simulink model "rfdc"  (R2019a)
settings: Solver=VariableStepAuto  StartTime=0.0  StopTime=10.0  RelTol=1e-3
libraries: xbsIndex_r4 x4
settings Model: Creator=mcb  LastModifiedBy=mcb

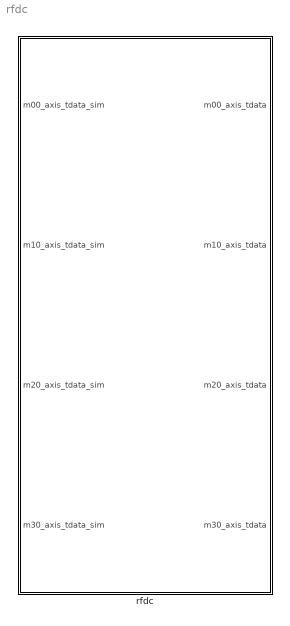
== system rfdc ==
  rfdc : Subsystem  Tag=xps:rfdc  mask(Xilinx RF Data Converter){Tile224_enable=on, Tile225_enable=on, Tile226_enable=on, Tile227_enable=on, enable_mts=off, sample_rate=2000, clk_out=250, enable_pll=on, ref_clk=250, axi_stream_clk=[], QT_adc0_enable=on, QT_adc0_digital_output=Real, QT_adc0_dec_mode=8x, QT_adc0_sample_per_cycle=1, QT_adc0_req_axis_clk=250, QT_adc0_mixer_type=Bypassed, QT_adc0_mixer_mode=Real -> Real, QT_adc0_nco_freq=0, QT_adc0_nco_phase=0, QT_adc0_coarse_freq=0, QT_adc0_nyquist_zone=Zone 1, QT_adc0_cal_mode=Mode 2, QT_adc1_enable=off, QT_adc1_digital_output=Real, QT_adc1_dec_mode=1x, QT_adc1_sample_per_cycle=4, QT_adc1_req_axis_clk=500, QT_adc1_mixer_type=Bypassed, QT_adc1_mixer_mode=Real -> Real, QT_adc1_nco_freq=0, QT_adc1_nco_phase=0, QT_adc1_coarse_freq=0, QT_adc1_nyquist_zone=Zone 2, QT_adc1_cal_mode=Mode 2, QT_adc2_enable=off, QT_adc2_digital_output=Real, QT_adc2_dec_mode=8x, QT_adc2_sample_per_cycle=1, QT_adc2_req_axis_clk=250, QT_adc2_mixer_type=Bypassed, QT_adc2_mixer_mode=Real -> Real, QT_adc2_nco_freq=0, QT_adc2_nco_phase=0, QT_adc2_coarse_freq=0, QT_adc2_nyquist_zone=Zone 1, QT_adc2_cal_mode=Mode 2, QT_adc3_enable=off, QT_adc3_digital_output=Real, QT_adc3_dec_mode=8x, QT_adc3_sample_per_cycle=1, QT_adc3_req_axis_clk=250, QT_adc3_mixer_type=Bypassed, QT_adc3_mixer_mode=Real -> Real, QT_adc3_nco_freq=0, QT_adc3_nco_phase=0, QT_adc3_coarse_freq=0, QT_adc3_nyquist_zone=Zone 1, QT_adc3_cal_mode=Mode 2, DT_adc0_enable=on, DT_adc0_digital_output=Real, DT_adc0_dec_mode=2x, DT_adc0_sample_per_cycle=8, DT_adc0_req_axis_clk=0, DT_adc0_mixer_type=Bypassed, DT_adc0_mixer_mode=Real -> Real, DT_adc0_nco_freq=0, DT_adc0_nco_phase=0, DT_adc0_coarse_freq=Fs/2, DT_adc0_nyquist_zone=Zone 1, DT_adc0_cal_mode=Mode 2, DT_adc1_enable=on, DT_adc1_digital_output=Real, DT_adc1_dec_mode=2x, DT_adc1_sample_per_cycle=8, DT_adc1_req_axis_clk=0, DT_adc1_mixer_type=Bypassed, DT_adc1_mixer_mode=Real -> Real, DT_adc1_nco_freq=0, DT_adc1_nco_phase=0, DT_adc1_coarse_freq=Fs/2, DT_adc1_nyquist_zone=Zone 1, DT_adc1_cal_mode=Mode 2}
      mask prompts: Tile224_enable "Tile 224"; Tile225_enable "Tile 225"; Tile226_enable "Tile 226"; Tile227_enable "Tile 227"; enable_mts "Enable Multi-Tile Sync"; sample_rate "Sampling Rate (Msps)"; clk_out "Clock Out (MHz)"; enable_pll "Enable Tile PLLs"; ref_clk "Reference Clock (MHz)"; axi_stream_clk "Required AXI4-Stream Clock (MHz)"; QT_adc0_enable "Enable ADC"; QT_adc0_digital_output "Digital Output Data"; QT_adc0_dec_mode "Decimation Mode"; QT_adc0_sample_per_cycle "Samples per AXI4-Stream Cycle"; QT_adc0_mixer_type "Mixer Type"; QT_adc0_mixer_mode "Mixer Mode"; QT_adc0_nco_freq "NCO Frequency (GHz)"; QT_adc0_nco_phase "NCO Phase"; QT_adc0_coarse_freq "Frequency"; QT_adc0_nyquist_zone "Nyquist Zone"; QT_adc0_cal_mode "Calibration Mode"; QT_adc1_enable "Enable ADC"; QT_adc1_digital_output "Digital Output Data"; QT_adc1_dec_mode "Decimation Mode"; QT_adc1_sample_per_cycle "Samples per AXI4-Stream Cycle"; QT_adc1_mixer_type "Mixer Type"; QT_adc1_mixer_mode "Mixer Mode"; QT_adc1_nco_freq "NCO Frequency (GHz)"; QT_adc1_nco_phase "NCO Phase"; QT_adc1_coarse_freq "Frequency"; QT_adc1_nyquist_zone "Nyquist Zone"; QT_adc1_cal_mode "Calibration Mode"; QT_adc2_enable "Enable ADC"; QT_adc2_digital_output "Digital Output Data"; QT_adc2_dec_mode "Decimation Mode"; QT_adc2_sample_per_cycle "Samples per AXI4-Stream Cycle"; QT_adc2_mixer_type "Mixer Type"; QT_adc2_mixer_mode "Mixer Mode"; QT_adc2_nco_freq "NCO Frequency (GHz)"; QT_adc2_nco_phase "NCO Phase"; QT_adc2_coarse_freq "Frequency"; QT_adc2_nyquist_zone "Nyquist Zone"; QT_adc2_cal_mode "Calibration Mode"; QT_adc3_enable "Enable ADC"; QT_adc3_digital_output "Digital Output Data"; QT_adc3_dec_mode "Decimation Mode"; QT_adc3_sample_per_cycle "Samples per AXI4-Stream Cycle"; QT_adc3_mixer_type "Mixer Type"; QT_adc3_mixer_mode "Mixer Mode"; QT_adc3_nco_freq "NCO Frequency (GHz)"; QT_adc3_nco_phase "NCO Phase"; QT_adc3_coarse_freq "Frequency"; QT_adc3_nyquist_zone "Nyquist Zone"; QT_adc3_cal_mode "Calibration Mode"; DT_adc0_enable "Enable ADC"; DT_adc0_digital_output "Digital Output Data"; DT_adc0_dec_mode "Decimation Mode"; DT_adc0_sample_per_cycle "Samples per AXI4-Stream Cycle"; DT_adc0_mixer_type "Mixer Type"; DT_adc0_mixer_mode "Mixer Mode"; DT_adc0_nco_freq "NCO Frequency (GHz)"; DT_adc0_nco_phase "NCO Phase"; DT_adc0_coarse_freq "Frequency"; DT_adc0_nyquist_zone "Nyquist Zone"; DT_adc0_cal_mode "Calibration Mode"; DT_adc1_enable "Enable ADC"; DT_adc1_digital_output "Digital Output Data"; DT_adc1_dec_mode "Decimation Mode"; DT_adc1_sample_per_cycle "Samples per AXI4-Stream Cycle"; DT_adc1_mixer_type "Mixer Type"; DT_adc1_mixer_mode "Mixer Mode"; DT_adc1_nco_freq "NCO Frequency (GHz)"; DT_adc1_nco_phase "NCO Phase"; DT_adc1_coarse_freq "Frequency"; DT_adc1_nyquist_zone "Nyquist Zone"; DT_adc1_cal_mode "Calibration Mode"
      mask help: CASPER RFDC
      mask init:
      | rfdc_mask(gcb);
      mask Help: eval('xlWeb([getenv(''MLIB_ROOT''), ''\doc\html\adc_zcu111\adc_zcu111.html''])')
      mask Callback Tile224_enable: enable_mts_opt(gcb);
      mask Callback sample_rate: update_rfdc_clocking(gcb);
      mask TypeOptions clk_out: 250 | 125 | 62.5 | 31.25
      mask Callback enable_pll:
      | %update_rfdc_clocking(gcb);
      | update_pll(gcb);
      mask TypeOptions ref_clk: 923.077 | 857.143 | 800 | 750 | 705.882 | 666.667 | 631.579 | 600 | 571.429 | 545.455 | 521.739 | 500 | 480 | 461.538 | 444.444 | 428.571 | 413.793 | 400 | 387.097 | 375 | 363.636 | 352.941 | 342.857 | 333.333 | 324.324 | 315.789 | 307.692 | 300 | 292.683 | 285.714 | 279.07 | 272.727 | 266.667 | 260.87 | 255.319 | 250 | 244.898 | 240 | 235.294 | 230.769 | 226.415 | 222.222 | 218.182 | 214.286 | 210.526 | 206.897 | 203.39 | 200 | 196.721 | 193.548 | 190.476 | 187.5 | 184.615 | 181.818 | 179.104 | 176.471 | 173.913 | 171.429 | 169.014 | 166.667 | 164.384 | 162.162 | 160 | 157.895 | 155.844 | 153.846 | 151.899 | 150 | 148.148 | 146.341 | 144.578 | 142.857 | 141.176 | 139.535 | 137.931 | 136.364 | 134.831 | 133.333 | 131.868 | 130.435 | 129.032 | 127.66 | 126.316 | 125 | 123.711 | 122.449 | 121.212 | 120 | 118.812 | 117.647 | 116.505 | 115.385 | 114.286 | 113.208 | 112.15 | 111.111 | 110.092 | 109.091 | 108.108 | 107.143 | 106.195 | 105.263 | 104.348 | 103.448 | 102.564
      mask Callback QT_adc0_enable: enable_adc_opt(gcb);
      mask TypeOptions QT_adc0_digital_output: Real | I/Q
      mask Callback QT_adc0_digital_output:
      | validate_digital_data(gcb);
      | update_axis_clk(gcb);
      mask TypeOptions QT_adc0_dec_mode: 1x | 2x | 4x | 8x
      mask Callback QT_adc0_dec_mode: update_axis_clk(gcb);
      mask TypeOptions QT_adc0_sample_per_cycle: 1 | 2 | 3 | 4 | 5 | 6 | 7 | 8 | 9 | 10 | 11 | 12
      mask Callback QT_adc0_sample_per_cycle:
      | %update_axis_clk(gcb);
      | update_axis_clk_label(gcb);
      mask TypeOptions QT_adc0_mixer_type: Bypassed
      mask Callback QT_adc0_mixer_type: mixertype_callback(gcb);
      mask TypeOptions QT_adc0_mixer_mode: Real -> Real
      mask Callback QT_adc0_mixer_mode: mixer_callback(gcb);
      mask TypeOptions QT_adc0_coarse_freq: 0
      mask TypeOptions QT_adc0_nyquist_zone: Zone 1 | Zone 2
      mask TypeOptions QT_adc0_cal_mode: Mode 1 | Mode 2
      mask Callback QT_adc1_enable: enable_adc_opt(gcb);
      mask TypeOptions QT_adc1_digital_output: Real | I/Q
      mask Callback QT_adc1_digital_output:
      | validate_digital_data(gcb);
      | update_axis_clk(gcb);
      mask TypeOptions QT_adc1_dec_mode: 1x | 2x | 4x | 8x
      mask Callback QT_adc1_dec_mode: update_axis_clk(gcb);
      mask TypeOptions QT_adc1_sample_per_cycle: 4 | 5 | 6 | 7 | 8 | 9 | 10 | 11 | 12
      mask Callback QT_adc1_sample_per_cycle: update_axis_clk_label(gcb);
      mask TypeOptions QT_adc1_mixer_type: Bypassed
      mask Callback QT_adc1_mixer_type: mixertype_callback(gcb);
      mask TypeOptions QT_adc1_mixer_mode: Real -> Real
      mask TypeOptions QT_adc1_coarse_freq: 0
      mask TypeOptions QT_adc1_nyquist_zone: Zone 1 | Zone 2
      mask TypeOptions QT_adc1_cal_mode: Mode 1 | Mode 2
      mask Callback QT_adc2_enable: enable_adc_opt(gcb);
      mask TypeOptions QT_adc2_digital_output: Real | I/Q
      mask Callback QT_adc2_digital_output:
      | validate_digital_data(gcb);
      | update_axis_clk(gcb);
      mask TypeOptions QT_adc2_dec_mode: 1x | 2x | 4x | 8x
      mask Callback QT_adc2_dec_mode: update_axis_clk(gcb);
      mask TypeOptions QT_adc2_sample_per_cycle: 1 | 2 | 3 | 4 | 5 | 6 | 7 | 8 | 9 | 10 | 11 | 12
      mask Callback QT_adc2_sample_per_cycle: update_axis_clk_label(gcb);
      mask TypeOptions QT_adc2_mixer_type: Bypassed
      mask Callback QT_adc2_mixer_type: mixertype_callback(gcb);
      mask TypeOptions QT_adc2_mixer_mode: Real -> Real
      mask TypeOptions QT_adc2_coarse_freq: 0
      mask TypeOptions QT_adc2_nyquist_zone: Zone 1 | Zone 2
      mask TypeOptions QT_adc2_cal_mode: Mode 1 | Mode 2
      mask Callback QT_adc3_enable: enable_adc_opt(gcb);
      mask TypeOptions QT_adc3_digital_output: Real | I/Q
      mask Callback QT_adc3_digital_output:
      | validate_digital_data(gcb);
      | update_axis_clk(gcb);
      mask TypeOptions QT_adc3_dec_mode: 1x | 2x | 4x | 8x
      mask Callback QT_adc3_dec_mode: update_axis_clk(gcb);
      mask TypeOptions QT_adc3_sample_per_cycle: 1 | 2 | 3 | 4 | 5 | 6 | 7 | 8 | 9 | 10 | 11 | 12
      mask Callback QT_adc3_sample_per_cycle: update_axis_clk_label(gcb);
      mask TypeOptions QT_adc3_mixer_type: Bypassed
      mask Callback QT_adc3_mixer_type: mixertype_callback(gcb);
      mask TypeOptions QT_adc3_mixer_mode: Real -> Real
      mask TypeOptions QT_adc3_coarse_freq: 0
      mask TypeOptions QT_adc3_nyquist_zone: Zone 1 | Zone 2
      mask TypeOptions QT_adc3_cal_mode: Mode 1 | Mode 2
      mask Callback DT_adc0_enable: enable_adc_opt(gcb);
      mask TypeOptions DT_adc0_digital_output: Real | I/Q
      mask Callback DT_adc0_digital_output:
      | validate_digital_data(gcb);
      | update_axis_clk(gcb);
      mask TypeOptions DT_adc0_dec_mode: 1x | 2x | 4x | 8x
      mask Callback DT_adc0_dec_mode: update_axis_clk(gcb);
      mask TypeOptions DT_adc0_sample_per_cycle: 1 | 2 | 3 | 4 | 5 | 6 | 7 | 8
      mask Callback DT_adc0_sample_per_cycle:
      | %update_axis_clk(gcb);
      | update_axis_clk_label(gcb);
      mask TypeOptions DT_adc0_mixer_type: Bypassed | Coarse | Fine
      mask Callback DT_adc0_mixer_type: mixertype_callback(gcb);
      mask TypeOptions DT_adc0_mixer_mode: Real -> Real | Real -> I/Q | I/Q -> I/Q
      mask Callback DT_adc0_mixer_mode: mixer_callback(gcb);
      mask TypeOptions DT_adc0_coarse_freq: Fs/2 | Fs/4 | -Fs/4
      mask TypeOptions DT_adc0_nyquist_zone: Zone 1 | Zone 2
      mask TypeOptions DT_adc0_cal_mode: Mode 1 | Mode 2
      mask Callback DT_adc1_enable: enable_adc_opt(gcb);
      mask TypeOptions DT_adc1_digital_output: Real | I/Q
      mask Callback DT_adc1_digital_output:
      | validate_digital_data(gcb);
      | update_axis_clk(gcb);
      mask TypeOptions DT_adc1_dec_mode: 1x | 2x | 4x | 8x
      mask Callback DT_adc1_dec_mode: update_axis_clk(gcb);
      mask TypeOptions DT_adc1_sample_per_cycle: 1 | 2 | 3 | 4 | 5 | 6 | 7 | 8
      mask Callback DT_adc1_sample_per_cycle:
      | %update_axis_clk(gcb);
      | update_axis_clk_label(gcb);
      mask TypeOptions DT_adc1_mixer_type: Bypassed | Coarse | Fine
      mask Callback DT_adc1_mixer_type: mixertype_callback(gcb);
      mask TypeOptions DT_adc1_mixer_mode: Real -> Real | Real -> I/Q | I/Q -> I/Q
      mask Callback DT_adc1_mixer_mode: mixer_callback(gcb);
      mask TypeOptions DT_adc1_coarse_freq: Fs/2 | Fs/4 | -Fs/4
      mask TypeOptions DT_adc1_nyquist_zone: Zone 1 | Zone 2
      mask TypeOptions DT_adc1_cal_mode: Mode 1 | Mode 2
      mask DialogControl TileSelect Prompt: ADC Tiles
      mask DialogControl pll_clocking_config_224 Prompt: Clocking and PLL Configuration
      mask DialogControl QuadTileConfig Prompt: Quad Tile Configuration
      mask DialogControl ADCPair01 Prompt: ADC Pair 0,1
      mask DialogControl QT_adc0 Prompt: ADC 0
      mask DialogControl QT_adc0_DataSettings Prompt: Data Settings
      mask DialogControl QT_adc0_req_axis_clk_label Prompt: Required AXI4-Stream clock:
      mask DialogControl QT_adc0_MixerSettings Prompt: MIxer Settings
      mask DialogControl QT_adc0_AnalogSettings Prompt: Analog Settings
      mask DialogControl QT_adc1 Prompt: ADC 1
      mask DialogControl QT_adc1_DataSettings Prompt: Data Settings
      mask DialogControl QT_adc1_req_axis_clk_label Prompt: Required AXI4-Stream clock:
      mask DialogControl QT_adc1_MixerSettings Prompt: MIxer Settings
      mask DialogControl QT_adc1_AnalogSettings Prompt: Analog Settings
      mask DialogControl ADCPair23 Prompt: ADC Pair 2,3
      mask DialogControl QT_adc2 Prompt: ADC 2
      mask DialogControl QT_adc2_DataSettings Prompt: Data Settings
      mask DialogControl QT_adc2_req_axis_clk_label Prompt: Required AXI4-Stream clock:
      mask DialogControl QT_adc2_MixerSettings Prompt: MIxer Settings
      mask DialogControl QT_adc2_AnalogSettings Prompt: Analog Settings
      mask DialogControl QT_adc3 Prompt: ADC 3
      mask DialogControl QT_adc3_DataSettings Prompt: Data Settings
      mask DialogControl QT_adc3_req_axis_clk_label Prompt: Required AXI4-Stream clock:
      mask DialogControl QT_adc3_MixerSettings Prompt: MIxer Settings
      mask DialogControl QT_adc3_AnalogSettings Prompt: Analog Settings
      mask DialogControl DualTileConfig Prompt: Dual Tile Configuration
      mask DialogControl DT_adc0 Prompt: ADC 0
      mask DialogControl DT_adc0_DataSettings Prompt: Data Settings
      mask DialogControl DT_adc0_req_axis_clk_label Prompt: Required AXI4-Stream clock:
      mask DialogControl DT_adc0_MixerSettings Prompt: MIxer Settings
      mask DialogControl DT_adc0_AnalogSettings Prompt: Analog Settings
      mask DialogControl DT_adc1 Prompt: ADC 1
      mask DialogControl DT_adc1_DataSettings Prompt: Data Settings
      mask DialogControl DT_adc1_req_axis_clk_label Prompt: Required AXI4-Stream clock:
      mask DialogControl DT_adc1_MixerSettings Prompt: MIxer Settings
      mask DialogControl DT_adc1_AnalogSettings Prompt: Analog Settings

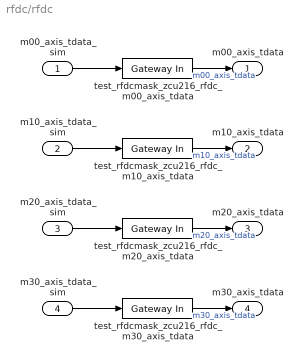
== system rfdc/rfdc ==
  m00_axis_tdata_sim : Inport
  m10_axis_tdata_sim : Inport  Port=2
  m20_axis_tdata_sim : Inport  Port=3
  m30_axis_tdata_sim : Inport  Port=4
  test_rfdcmask_zcu216_rfdc_m00_axis_tdata : xbsIndex_r4/Gateway In  gui_display_data_type=Fixed-point  arith_type="Signed  (2's comp)"  n_bits=16  bin_pt=0  preci_type=Single  exp_width=8  frac_width=24  rows=1  columns=1  quantization="Round  (unbiased: +/- Inf)"  overflow=Saturate  period=1  UseAsADC=off  ADCChannel='1'  interface=None  automatic_assignment=on  address_offset=hex2dec('00')  intf_name=''  intf_description=''  default_value=0  timing_constraint=None  locs_specified=off  LOCs={}  io_standard={}  inherit_from_input=off  hdl_port=on  dbl_ovrd=off  block_type=gatewayin
  test_rfdcmask_zcu216_rfdc_m10_axis_tdata : xbsIndex_r4/Gateway In  gui_display_data_type=Fixed-point  arith_type="Signed  (2's comp)"  n_bits=16  bin_pt=0  preci_type=Single  exp_width=8  frac_width=24  rows=1  columns=1  quantization="Round  (unbiased: +/- Inf)"  overflow=Saturate  period=1  UseAsADC=off  ADCChannel='1'  interface=None  automatic_assignment=on  address_offset=hex2dec('00')  intf_name=''  intf_description=''  default_value=0  timing_constraint=None  locs_specified=off  LOCs={}  io_standard={}  inherit_from_input=off  hdl_port=on  dbl_ovrd=off  block_type=gatewayin
  test_rfdcmask_zcu216_rfdc_m20_axis_tdata : xbsIndex_r4/Gateway In  gui_display_data_type=Fixed-point  arith_type="Signed  (2's comp)"  n_bits=16  bin_pt=0  preci_type=Single  exp_width=8  frac_width=24  rows=1  columns=1  quantization="Round  (unbiased: +/- Inf)"  overflow=Saturate  period=1  UseAsADC=off  ADCChannel='1'  interface=None  automatic_assignment=on  address_offset=hex2dec('00')  intf_name=''  intf_description=''  default_value=0  timing_constraint=None  locs_specified=off  LOCs={}  io_standard={}  inherit_from_input=off  hdl_port=on  dbl_ovrd=off  block_type=gatewayin
  test_rfdcmask_zcu216_rfdc_m30_axis_tdata : xbsIndex_r4/Gateway In  gui_display_data_type=Fixed-point  arith_type="Signed  (2's comp)"  n_bits=16  bin_pt=0  preci_type=Single  exp_width=8  frac_width=24  rows=1  columns=1  quantization="Round  (unbiased: +/- Inf)"  overflow=Saturate  period=1  UseAsADC=off  ADCChannel='1'  interface=None  automatic_assignment=on  address_offset=hex2dec('00')  intf_name=''  intf_description=''  default_value=0  timing_constraint=None  locs_specified=off  LOCs={}  io_standard={}  inherit_from_input=off  hdl_port=on  dbl_ovrd=off  block_type=gatewayin
  m00_axis_tdata : Outport  VectorParamsAs1DForOutWhenUnconnected=off
  m10_axis_tdata : Outport  Port=2  VectorParamsAs1DForOutWhenUnconnected=off
  m20_axis_tdata : Outport  Port=3  VectorParamsAs1DForOutWhenUnconnected=off
  m30_axis_tdata : Outport  Port=4  VectorParamsAs1DForOutWhenUnconnected=off
  wires:
  m00_axis_tdata_sim/1 -> test_rfdcmask_zcu216_rfdc_m00_axis_tdata/1
  test_rfdcmask_zcu216_rfdc_m00_axis_tdata/1 -> m00_axis_tdata/1  "m00_axis_tdata"
  m10_axis_tdata_sim/1 -> test_rfdcmask_zcu216_rfdc_m10_axis_tdata/1
  test_rfdcmask_zcu216_rfdc_m10_axis_tdata/1 -> m10_axis_tdata/1  "m10_axis_tdata"
  m20_axis_tdata_sim/1 -> test_rfdcmask_zcu216_rfdc_m20_axis_tdata/1
  test_rfdcmask_zcu216_rfdc_m20_axis_tdata/1 -> m20_axis_tdata/1  "m20_axis_tdata"
  m30_axis_tdata_sim/1 -> test_rfdcmask_zcu216_rfdc_m30_axis_tdata/1
  test_rfdcmask_zcu216_rfdc_m30_axis_tdata/1 -> m30_axis_tdata/1  "m30_axis_tdata"
